simulink model "test_CO_bump"  (R2012b)
settings: Solver=FixedStepDiscrete  StartTime=0.0  StopTime=Inf  FixedStep=.001  RelTol=1e-3
libraries: simulink x4
CloseFcn:
  | rtwprivate ssgencode ModelCloseRequest rwalk_multi_local_v1
settings Model: ParamWorkspaceSource=ReferencedWorkspace  ExtModeArmWhenConnect=off  BufferReuse=off  Creator=limblab  LastModifiedBy=limblab
settings DataIOCC: LimitDataPoints=off  SaveFormat=StructureWithTime  SignalLoggingSaveFormat=ModelDataLogs  SaveState=on  SignalLoggingName=sigsOut
settings OptimizationCC: BlockReduction=off  BooleanDataType=off  OptimizeBlockIOStorage=off  BufferReuse=off  ExpressionFolding=off  FoldNonRolledExpr=off  LocalBlockOutputs=off  InitFltsAndDblsToZero=on
settings DebuggingCC: SaveWithParameterizedLinksMsg=none  SignalResolutionControl=TryResolveAllWithWarning  SolverPrmCheckMsg=none  MultiTaskDSMMsg=warning  MultiTaskCondExecSysMsg=none  FcnCallInpInsideContextMsg=UseLocalSettings  StrictBusMsg=None
settings HardwareCC: ProdIntDivRoundTo=Zero  ProdEndianess=LittleEndian  ProdHWDeviceType=Generic->32-bit x86 compatible  TargetIntDivRoundTo=Zero  TargetEndianess=LittleEndian  TargetHWDeviceType=32-bit xPC Target (Intel Pentium)
settings SFSimCC: SimParseCustomCode=off
settings RTWCC: SystemTargetFile=xpctarget.tlc  TemplateMakefile=xpc_default_tmf  Description=xPC Target  GenerateReport=on  ProcessScript=xpctarget_make_rtw_hook  IncludeERTFirstTime=on
settings xpcTargetCC: TargetFcnLib=ansi_tfl_tmw.mat  CodeReplacementLibrary=XPC_BLAS  ParMdlRefBuildCompliant=on  ConcurrentExecutionCompliant=on  CombineSignalStateStructs=off  GRTInterface=on  xPCTaskExecutionProfile=off  xPCRL32EventNumber=5000  xPCisDownloadable=off  xPCLoadParamSetFile=off  xPCConcurrentTasks=off  xPCEnableSFAnimation=off

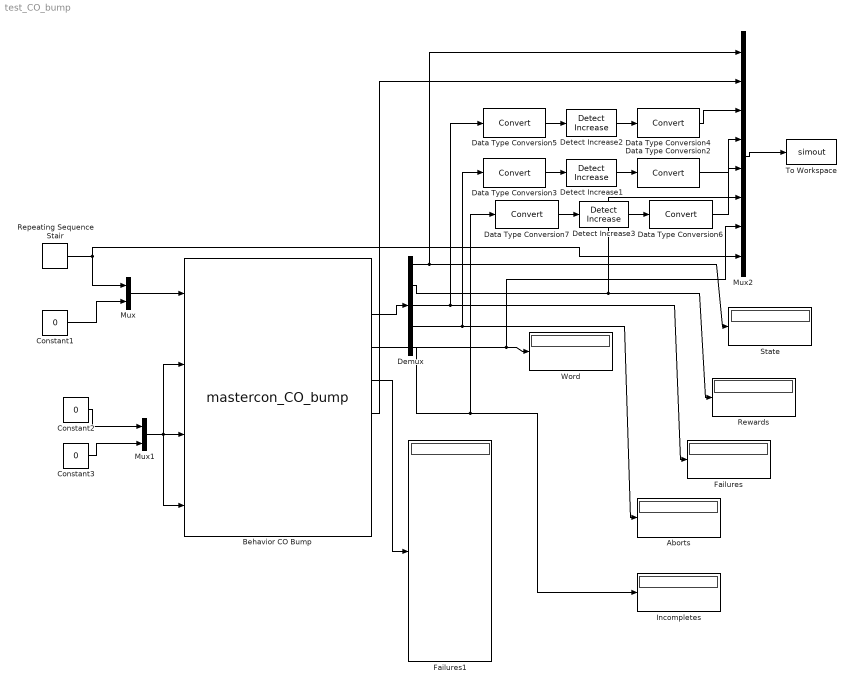
== system test_CO_bump ==
  Aborts : Display
  Behavior CO Bump : S-Function  FunctionName=mastercon_CO_bump  Parameters=0 0 4 10 0 2 .3 .05 .75 .3 .4 .5 0 .5 1 0 360 45 0 .5 1 .75 1  EnableBusSupport=off
      mask Display:
      | disp('Master Control')
      | port_label('input',1,'pos')
      | port_label('input',2,'offsets')
      | port_label('input',3,'force')
      | port_label('input',4,'catch force')
      | port_label('output',1,'force')
      | port_label('output',2,'status')
      | port_label('output',3,'word')
      | port_label('output',4,'targets')
      | port_label('output',5,'reward')
      | port_label('output',6,'tone')
      | port_label('output',7,'version')
      | port_label('output',8,'pos')
  Constant1 : Constant  Value=0
  Constant2 : Constant  Value=0
  Constant3 : Constant  Value=0
  Data Type Conversion{2..7} (6 alike) : DataTypeConversion
  Demux : Demux  Outputs=5
  Detect Increase1 : simulink/Logic and Bit Operations/Detect Increase  vinit=0.0  InputProcessing=Inherited  OutDataTypeStr=uint8
  Detect Increase2 : simulink/Logic and Bit Operations/Detect Increase  vinit=0.0  InputProcessing=Inherited  OutDataTypeStr=uint8
  Detect Increase3 : simulink/Logic and Bit Operations/Detect Increase  vinit=0.0  InputProcessing=Inherited  OutDataTypeStr=uint8
  Failures : Display
  Failures1 : Display
  Incompletes : Display
  Mux : Mux  Inputs=2
  Mux1 : Mux  Inputs=2
  Mux2 : Mux  Inputs=8
  Repeating Sequence Stair : simulink/Sources/Repeating Sequence Stair  OutValues=[0 -10 0 0 10 0].'  tsamp=.001  OutMin=[]  OutMax=[]  OutDataTypeStr=float('double')  OutputDataTypeScalingMode=Specify via dialog  OutDataType=float('double')  ConRadixGroup=Best Precision: Vector-wise  OutScaling=2^-12
  Rewards : Display
  State : Display
  To Workspace : ToWorkspace  VariableName=simout  SampleTime=-1  SaveFormat=Structure
  Word : Display
  wires:
  Constant1/1 -> Mux/2
  Mux/1 -> Behavior CO Bump/1
  Behavior CO Bump/2 -> Demux/1
  Demux/1 -> State/1, Mux2/1
  Constant2/1 -> Mux1/1
  Constant3/1 -> Mux1/2
  Mux1/1 -> Behavior CO Bump/4, Behavior CO Bump/2, Behavior CO Bump/3
  Demux/2 -> Rewards/1, Mux2/6
  Demux/3 -> Failures/1, Data Type Conversion5/1
  Behavior CO Bump/4 -> Failures1/1
  Demux/5 -> Incompletes/1, Data Type Conversion7/1
  Demux/4 -> Aborts/1, Data Type Conversion3/1
  Mux2/1 -> To Workspace/1
  Data Type Conversion3/1 -> Detect Increase1/1
  Detect Increase1/1 -> Data Type Conversion2/1
  Data Type Conversion5/1 -> Detect Increase2/1
  Detect Increase2/1 -> Data Type Conversion4/1
  Data Type Conversion4/1 -> Mux2/3
  Data Type Conversion2/1 -> Mux2/4
  Data Type Conversion7/1 -> Detect Increase3/1
  Detect Increase3/1 -> Data Type Conversion6/1
  Data Type Conversion6/1 -> Mux2/5
  Behavior CO Bump/5 -> Mux2/2
  Repeating Sequence Stair/1 -> Mux/1, Mux2/8
  Behavior CO Bump/3 -> Mux2/7, Word/1
